simulink model "inv_dynR2018a"  (R2018a)
settings: Solver=ode23  StartTime=0.0  StopTime=5  FixedStep=.001  MaxStep=.1  RelTol=1e-3
settings Model: Creator=imi  LastModifiedBy=SINA
settings CodeAppCC: StateflowObjectComments=on

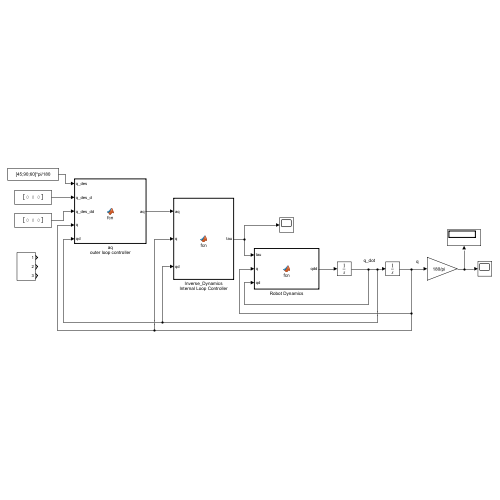
[thumbnail: Simulink's stored preview of the top-level diagram]
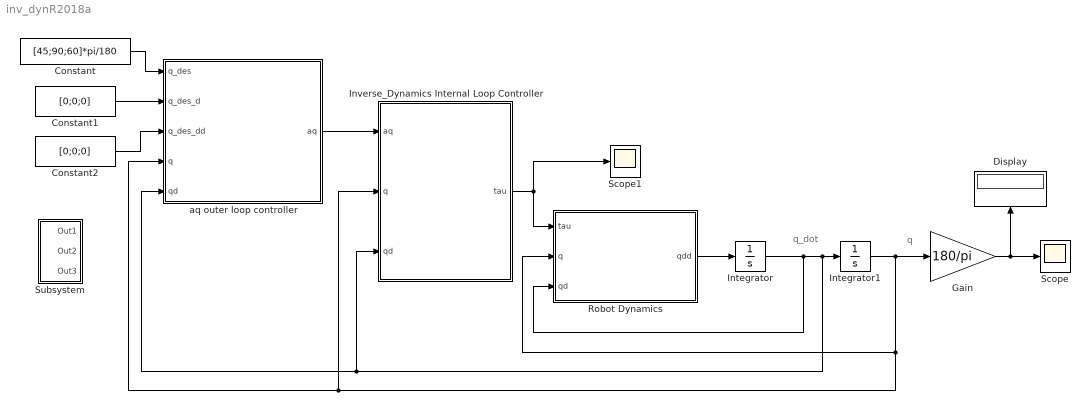
== system inv_dynR2018a ==
  note: q
  note: q_dot
  Constant : Constant  Value=[45;90;60]*pi/180
  Constant1 : Constant  Value=[0;0;0]
  Constant2 : Constant  Value=[0;0;0]
  Display : Display
  Gain : Gain  Gain=180/pi
  Integrator : Integrator  InitialCondition=zeros(3,1)
  Integrator1 : Integrator  InitialCondition=[45;95;95]*pi/180*0
  Inverse_Dynamics Internal Loop Controller : MATLAB Function  TreatAsAtomicUnit=on
  Robot Dynamics : MATLAB Function  TreatAsAtomicUnit=on
  Scope : Scope
  Scope1 : Scope
  Subsystem : Subsystem
  aq outer loop controller : MATLAB Function  TreatAsAtomicUnit=on
  wires:
  Integrator/1 -> Robot Dynamics/3(qd), aq outer loop controller/5(qd), Inverse_Dynamics Internal Loop Controller/3(qd), Integrator1/1
  Robot Dynamics/1(qdd) -> Integrator/1
  Integrator1/1 -> aq outer loop controller/4(q), Inverse_Dynamics Internal Loop Controller/2(q), Robot Dynamics/2(q), Gain/1
  Inverse_Dynamics Internal Loop Controller/1(tau) -> Robot Dynamics/1(tau), Scope1/1
  Gain/1 -> Scope/1, Display/1
  Constant/1 -> aq outer loop controller/1(q_des)
  Constant1/1 -> aq outer loop controller/2(q_des_d)
  Constant2/1 -> aq outer loop controller/3(q_des_dd)
  aq outer loop controller/1(aq) -> Inverse_Dynamics Internal Loop Controller/1(aq)

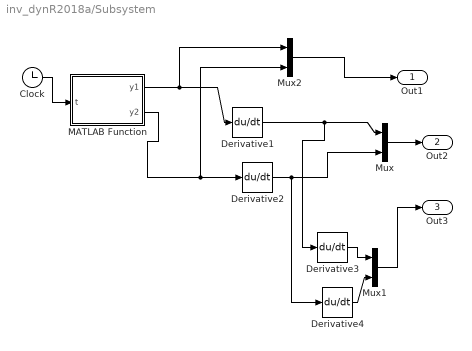
== system inv_dynR2018a/Subsystem ==
  Clock : Clock
  Derivative{1..4} (4 alike) : Derivative
  MATLAB Function : MATLAB Function  TreatAsAtomicUnit=on
  Mux : Mux  Inputs=2
  Mux1 : Mux  Inputs=2
  Mux2 : Mux  Inputs=2
  Out1 : Outport
  Out2 : Outport  Port=2
  Out3 : Outport  Port=3
  wires:
  Clock/1 -> MATLAB Function/1(t)
  Derivative2/1 -> Derivative4/1, Mux/2
  MATLAB Function/2(y2) -> Mux2/2, Derivative2/1
  Derivative1/1 -> Derivative3/1, Mux/1
  MATLAB Function/1(y1) -> Mux2/1, Derivative1/1
  Mux1/1 -> Out3/1
  Mux/1 -> Out2/1
  Derivative3/1 -> Mux1/1
  Derivative4/1 -> Mux1/2
  Mux2/1 -> Out1/1

== matlab function inv_dynR2018a/Inverse_Dynamics Internal Loop Controller ==
  data: aq input; q input; qd input; tau output
function tau = fcn(aq,q,qd)

q1=q(1);
q2=q(2);
q3=q(3);

q1d=qd(1);
q2d=qd(2);
q3d=qd(3);

%%%%%%%%%%%%%%Estimation

g=9.81;
%% D matrix
a1 = 3711123.19;
a2 = 596800.7545;
a3 = 331555.9747;
a4 = 53642.39711;
a5 = 634939.518;
a6 = 2803935.578;
a7 = 2828662.354;
a8 = 99466.79242;
a9 = 100433.5775;
a10 = 10959503.36;
a11 = 938582.3772;
a12 = 1193601.509;
a13 = 36757.08547;

b1 = 0.9129049856;
b2 = 0.4488127224;
b3 = 0.8976254448;
b4 = 0.5470269195;
b5 = 0.09795560006;
b6 = 0.05116245311;
b7 = 1.121983604;
b8 = 1.220635142;
b9 = 0.3985389635;
b10 = 1.181241563;

c1 = 11134263.19;
c2 = 301181.5542;

d11=a1*cos(q2+b1)-a2*cos(q3+b2)-a3*cos(q2+q3+b2)+a4*cos(2*q2+2*q3+b3)+a5*cos(2*q2+b4)-a2*cos(2*q2+q3+b2)+c1;
d12=a6*cos(q1+b5)+a7*cos(q2+b6)+a8*cos(q2+q3-b7);
d13=a8*cos(q2+q3-b7)-a9*cos(q1+b8);
d22=a10-a11*cos(2*q1-b9)-a12*cos(q3+b2);
d23=a13*cos(2*q1+b10)-a2*cos(q3+b2)+c2;
d33=a13*cos(2*q1+b10)+c2;

%% C matrix
h1=a13*cos(2*q1-0.3895547636);
h2=a11*sin(2*q1-b9);
h3=a2*sin(q3+b2);
h4=a2*sin(2*q2+q3+b2);
h5=298400.3773*cos(2*q2+q3-b7);
h6=a4*cos(2*q2+2*q3-0.673170882);
h7=a8*cos(q2+q3+b2);
h8=165777.9874*sin(q2+q3+b2);
h9=165777.9874*cos(q2+q3-b7);
h10=1855561.595*cos(0.6578913412-q2);
h11=298400.3773*cos(b7-q3);
h12=a5*sin(2*q2+b4);

c111=0;
c121=h8-h6-h10-h12+h4;
c131=h5-h6+h11+h9;
c221=h7-h2-a7*cos(1.5196339-q2);
c231=h7+h1;
c331=c231;

c112=h6-a6*sin(q1+b5)-h8+h10+h12-h4;
c122=h2;
c132=-h1;
c222=0;
c232=h3;
c332=h3;

c113=h6-h5-h11+a9*cos(q1-0.3501611849)-h9;
c123=-h1;
c133=-h1;
c223=-h3;
c233=0;
c333=0;



% 
M_hat=[d11,d12,d13;d12,d22,d23;d13,d23,d33];
%C_hat=[c111*q1d+c211*q2d+c311*q3d,c121*q1d+c221*q2d+c321*q3d,c131*q1d+c231*q2d+c331*q3d;
%    c112*q1d+c212*q2d+c312*q3d,c122*q1d+c222*q2d+c322*q3d,c132*q1d+c232*q2d+c332*q3d;
%    c113*q1d+c213*q2d+c313*q3d,c123*q1d+c223*q2d+c323*q3d,c133*q1d+c233*q2d+c333*q3d]
C_hat=[c121*q2d+c131*q3d,c121*q1d+c221*q2d+c231*q3d,c131*q1d+c231*q2d+c331*q3d;
   c112*q1d+c122*q2d+c132*q3d,c122*q1d+c232*q3d,c132*q1d+c232*q2d+c332*q3d;
   c113*q1d+c123*q2d+c133*q3d,c123*q1d+c223*q2d+c233*q3d,c133*q1d];
G_hat=[0;21618.172345*cos(q2+q3+b2)-241973.322224*cos(q2+0.91290498);21618.172345*cos(q2+q3+b2)];


%%%%%%%%%%%%%%%%%%%%%%%%%%%%%%%%%%%%%%%%%%%%%%%%%%%%%%%%%%%%%%%%%%%%%%%%%
tau=M_hat*aq+C_hat*qd+G_hat;

== matlab function inv_dynR2018a/Robot Dynamics ==
  data: tau input; q input; qdd output; qd input
function qdd = fcn(tau,q,qd)

q1=q(1);
q2=q(2);
q3=q(3);

q1d=qd(1);
q2d=qd(2);
q3d=qd(3);

%%%%%%%%%%%%%%Estimation

g=9.81;
%% D matrix
a1 = 3711123.19;
a2 = 596800.7545;
a3 = 331555.9747;
a4 = 53642.39711;
a5 = 634939.518;
a6 = 2803935.578;
a7 = 2828662.354;
a8 = 99466.79242;
a9 = 100433.5775;
a10 = 10959503.36;
a11 = 938582.3772;
a12 = 1193601.509;
a13 = 36757.08547;

b1 = 0.9129049856;
b2 = 0.4488127224;
b3 = 0.8976254448;
b4 = 0.5470269195;
b5 = 0.09795560006;
b6 = 0.05116245311;
b7 = 1.121983604;
b8 = 1.220635142;
b9 = 0.3985389635;
b10 = 1.181241563;

c1 = 11134263.19;
c2 = 301181.5542;

d11=a1*cos(q2+b1)-a2*cos(q3+b2)-a3*cos(q2+q3+b2)+a4*cos(2*q2+2*q3+b3)+a5*cos(2*q2+b4)-a2*cos(2*q2+q3+b2)+c1;
d12=a6*cos(q1+b5)+a7*cos(q2+b6)+a8*cos(q2+q3-b7);
d13=a8*cos(q2+q3-b7)-a9*cos(q1+b8);
d22=a10-a11*cos(2*q1-b9)-a12*cos(q3+b2);
d23=a13*cos(2*q1+b10)-a2*cos(q3+b2)+c2;
d33=a13*cos(2*q1+b10) +c2;

%% C matrix
h1=a13*cos(2*q1-0.3895547636);
h2=a11*sin(2*q1-b9);
h3=a2*sin(q3+b2);
h4=a2*sin(2*q2+q3+b2);
h5=298400.3773*cos(2*q2+q3-b7);
h6=a4*cos(2*q2+2*q3-0.673170882);
h7=a8*cos(q2+q3+b2);
h8=165777.9874*sin(q2+q3+b2);
h9=165777.9874*cos(q2+q3-b7);
h10=1855561.595*cos(0.6578913412-q2);
h11=298400.3773*cos(b7-q3);
h12=a5*sin(2*q2+b4);

c111=0;
c121=h8-h6-h10-h12+h4;
c131=h5-h6+h11+h9;
c221=h7-h2-a7*cos(1.5196339-q2);
c231=h7+h1;
c331=c231;

c112=h6-a6*sin(q1+b5)-h8+h10+h12-h4;
c122=h2;
c132=-h1;
c222=0;
c232=h3;
c332=h3;

c113=h6-h5-h11+a9*cos(q1-0.3501611849)-h9;
c123=-h1;
c133=-h1;
c223=-h3;
c233=0;
c333=0;



% 
M=[d11,d12,d13;d12,d22,d23;d13,d23,d33];
%C=[c111*q1d+c211*q2d+c311*q3d,c121*q1d+c221*q2d+c321*q3d,c131*q1d+c231*q2d+c331*q3d;
%    c112*q1d+c212*q2d+c312*q3d,c122*q1d+c222*q2d+c322*q3d,c132*q1d+c232*q2d+c332*q3d;
%    c113*q1d+c213*q2d+c313*q3d,c123*q1d+c223*q2d+c323*q3d,c133*q1d+c233*q2d+c333*q3d]
C=[c121*q2d+c131*q3d,c121*q1d+c221*q2d+c231*q3d,c131*q1d+c231*q2d+c331*q3d;
   c112*q1d+c122*q2d+c132*q3d,c122*q1d+c232*q3d,c132*q1d+c232*q2d+c332*q3d;
   c113*q1d+c123*q2d+c133*q3d,c123*q1d+c223*q2d+c233*q3d,c133*q1d];
G=[0;21618.172345*cos(q2+q3+b2)-241973.322224*cos(q2+0.91290498);21618.172345*cos(q2+q3+b2)];



qdd=pinv(M)*(tau-C*qd-G);

== matlab function inv_dynR2018a/Subsystem/MATLAB Function ==
  data: t input; y1 output; y2 output
function [y1,y2]= fcn(t)

y1=sin(.1*t);
y2=sin(.05*t+pi/6);

== matlab function inv_dynR2018a/aq outer loop controller ==
  data: q_des input; q_des_d input; q_des_dd input; q input; qd input; aq output
function aq = fcn(q_des,q_des_d,q_des_dd,q,qd)

q1=q(1);
q2=q(2);
q3=q(3);

q1d=qd(1);
q2d=qd(2);
q3d=qd(3);





q_tilde=q-q_des;
q_tilde_d=qd-q_des_d;


zita=1;
wn=2*pi*3;

K1=eye(3)*2*zita*wn;
K0=eye(3)*wn^2;


B=[zeros(3,3);eye(3)];
e=[q_tilde;q_tilde_d];
P=eye(6);
rho=.1;


if norm(B'*P*e)~=0
    delta=-rho*(B'*P*e)/norm(B'*P*e);
else
    delta=zeros(3,1);
end

%delta=0*delta;

aq=q_des_dd-K0*q_tilde-K1*q_tilde_d+delta;%external loop
